simulink model "Report_12"  (R2022a)
settings: Solver=VariableStepAuto  StartTime=0.0  StopTime=1  RelTol=1e-3
settings Model: Creator=takahiro  LastModifiedBy=takahiro

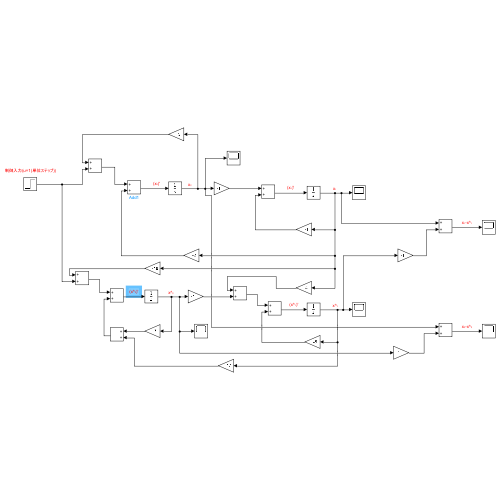
[thumbnail: Simulink's stored preview of the top-level diagram]
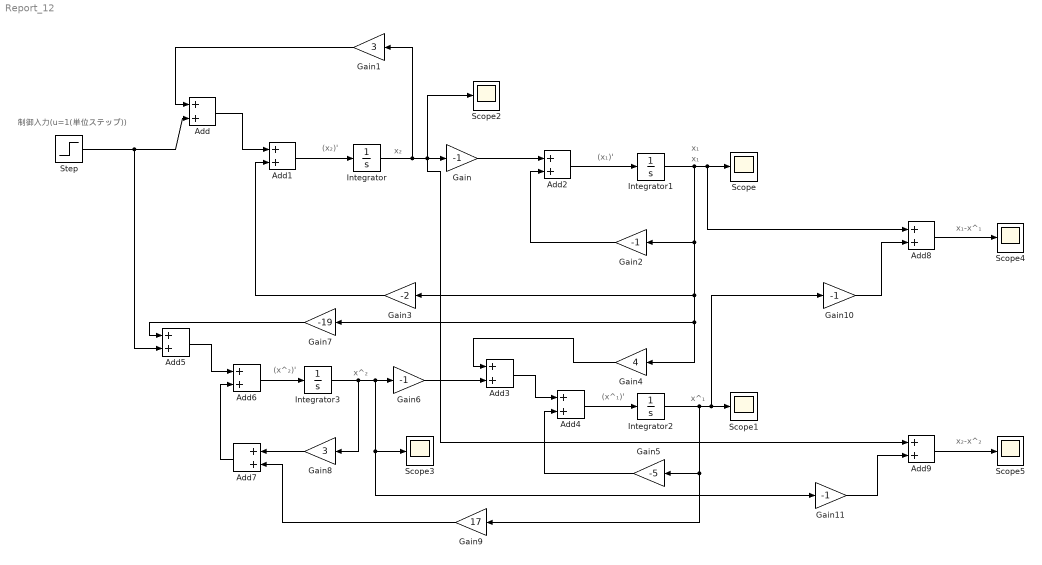
== system Report_12 ==
  note: x₂
  note: 制御入力(u=1(単位ステップ))
  note: (x₂)'
  note: (x₁)'
  note: x₁
  note: (x^₂)'
  note: x^₂
  note: (x^₁)'
  note: x^₁
  note: x₁-x^₁
  note: x₂-x^₂
  note: x₁
  Add{,1..9} (10 alike) : Sum
  Gain{,2,6,10..11} (5 alike) : Gain  Gain=-1
  Gain1 : Gain  Gain=3
  Gain3 : Gain  Gain=-2
  Gain4 : Gain  Gain=4
  Gain5 : Gain  Gain=-5
  Gain7 : Gain  Gain=-19
  Gain8 : Gain  Gain=3
  Gain9 : Gain  Gain=17
  Integrator{,1..3} (4 alike) : Integrator
  Scope{,1..5} (6 alike) : Scope
  Step : Step  Before=1  SampleTime=0
  wires:
  Step/1 -> Add5/2, Add/2
  Add/1 -> Add1/1
  Add1/1 -> Integrator/1
  Integrator/1 -> Gain1/1, Add9/1, Gain/1, Scope2/1
  Gain1/1 -> Add/1
  Gain/1 -> Add2/1
  Add2/1 -> Integrator1/1
  Integrator1/1 -> Gain3/1, Gain7/1, Gain4/1, Gain2/1, Add8/1, Scope/1
  Gain2/1 -> Add2/2
  Gain3/1 -> Add1/2
  Integrator2/1 -> Gain9/1, Gain5/1, Gain10/1, Scope1/1
  Gain4/1 -> Add3/1
  Add3/1 -> Add4/1
  Add4/1 -> Integrator2/1
  Gain5/1 -> Add4/2
  Gain6/1 -> Add3/2
  Integrator3/1 -> Gain8/1, Gain11/1, Scope3/1, Gain6/1
  Gain7/1 -> Add5/1
  Add5/1 -> Add6/1
  Add6/1 -> Integrator3/1
  Gain8/1 -> Add7/1
  Add7/1 -> Add6/2
  Gain9/1 -> Add7/2
  Gain10/1 -> Add8/2
  Add8/1 -> Scope4/1
  Gain11/1 -> Add9/2
  Add9/1 -> Scope5/1
